simulink model "adc_pdb_trigger_s32k14x"  (Simulink 9.2)
settings: Solver=FixedStepDiscrete  StartTime=0.0  StopTime=10.0  FixedStep=0.1  RelTol=1e-3  EnableMultiTasking=on
InitFcn:
  | mbd_s32k_consistency_checks(bdroot(gcs));
undefined symbols (not defined in the file): LQFP
libraries: mbd_s32k1xx_ec_toolbox x10, simulink x1
Description:
  | This example demonstrates using of ADC module in hardware trigger mode
  | for measuring a signal from AD12 channel (potentiometer) and AD6 channel
  | (temperature)
  | 
  | Validation:
  | - Use adc_pdb_trigger_s32k14x.pmp to validate the ADC conversion
settings Model: Creator=NXP MBDT Team  LastModifiedBy=shivama
settings DataIOCC: ExternalInput=off  InitialState=off  SignalLoggingSaveFormat=Dataset  SaveOutput=off  SignalLogging=off  SaveTime=off
settings OptimizationCC: DefaultParameterBehavior=Inlined  PassReuseOutputArgsAs=Individual arguments  LifeSpan=auto
settings DebuggingCC: SolverPrmCheckMsg=warning  InheritedTsInSrcMsg=none  SingleTaskRateTransMsg=error  ParameterTunabilityLossMsg=error  FcnCallInpInsideContextMsg=error  UnconnectedInputMsg=error  UnconnectedOutputMsg=error  UnconnectedLineMsg=error  AllowSymbolicDim=off  UnknownTsInhSupMsg=error
settings HardwareCC: ProdLargestAtomicInteger=Long  ProdLargestAtomicFloat=Double  ProdEndianess=LittleEndian  ProdHWDeviceType=ARM Compatible->ARM Cortex
settings SFSimCC: MATLABDynamicMemAlloc=off
settings RTWCC: SystemTargetFile=mbd_s32k.tlc  MakeCommand=mbd_s32k_make_rtw COPY_MDLREF_INCLUDES=0  TemplateMakefile=mbd_s32k.tmf  Description=Model Based Design Toolbox S32K14x Code Generation Target  GenerateReport=on  IncludeHyperlinkInReport=on  LaunchReport=on  GenerateTraceInfo=on  GenerateTraceReport=on  GenerateTraceReportSl=on  GenerateTraceReportSf=on  GenerateTraceReportEml=on
settings CodeAppCC: ForceParamTrailComments=on  IgnoreCustomStorageClasses=off  OperatorAnnotations=on  SimulinkDataObjDesc=on  SFDataObjDesc=on  InsertBlockDesc=on  StateflowObjectComments=off
settings STFCustomTargetCC: MultiwordLength=256  ModelReferenceCompliant=off  CombineOutputUpdateFcns=on  ERTCustomFileBanners=on  SupportContinuousTime=off  SupportNonInlinedSFcns=off  RemoveResetFunc=on  MATLABClassNameForMDSCustomization=Simulink.SoftwareTarget.ERTCustomization  GRTInterface=off  SystemTargetFile=mbd_s32k.tlc
settings ERTTargetCC: ModelReferenceCompliant=off  ParMdlRefBuildCompliant=off  CompOptLevelCompliant=off  ConcurrentExecutionCompliant=off  ModelStepFunctionPrototypeControlCompliant=off  CPPClassGenCompliant=off  UseToolchainInfoCompliant=off  InlinedParameterPlacement=NonHierarchical  ERTCustomFileTemplate=example_file_process.tlc

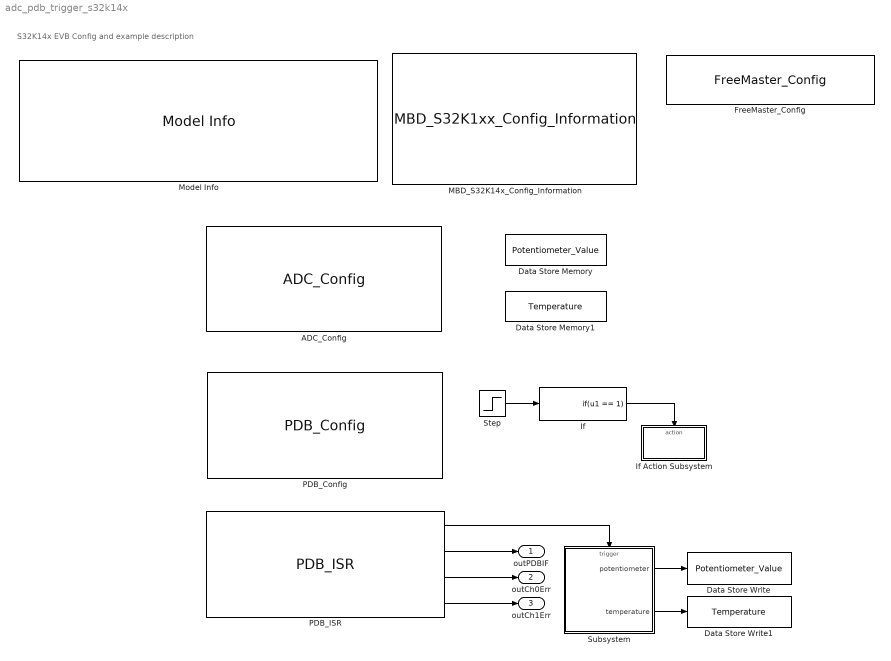
== system adc_pdb_trigger_s32k14x ==
  note: S32K14x EVB Config and example description
  ADC_Config : mbd_s32k1xx_ec_toolbox/Motor Control Blocks/ADC Blocks/ADC_Config  Priority=1  instance=0  mode=12-bit conversion  smplts=29  adiclk=alternate clock 1  adiv=input clock  show_adv_opts=on  pretrgsel=PDB pre-trigger  swpretrg=Disabled  adtrg=hardware  trgsel=PDB output  refsel=Vrefh and Vrefl  supply_monitoring=off  acfe=off  acfgt=off  acren=off  cv1=0  cv2=0  adco=off  avge=off  avgs=4 samples
  Data Store Memory : DataStoreMemory  DataStoreName=Potentiometer_Value  ReadBeforeWriteMsg=warning  WriteAfterWriteMsg=warning  WriteAfterReadMsg=warning  ShowAdditionalParam=off  OutDataTypeStr=uint32
  Data Store Memory1 : DataStoreMemory  DataStoreName=Temperature  ReadBeforeWriteMsg=warning  WriteAfterWriteMsg=warning  WriteAfterReadMsg=warning  ShowAdditionalParam=off  OutDataTypeStr=uint32
  Data Store Write : DataStoreWrite  DataStoreName=Potentiometer_Value
  Data Store Write1 : DataStoreWrite  DataStoreName=Temperature
  FreeMaster_Config : mbd_s32k1xx_ec_toolbox/Utility Blocks/FreeMaster_Config  interface=LPUART1  baudrate=115200  rxd=PTC6: [LPUART1_RX | Receive]  txd=PTC7: [LPUART1_TX | Transmit]  mode=Short Interrupt  isr_prio=15  show_adv_opts=off  use_scope=on  max_scope_vars=8  use_recorder=on  max_rec_vars=8  rec_buff_size=1024  rec_timebase=0 milliseconds  comm_buffer_size_auto=on  comm_buffer_size=255  comm_rqueue_size_default=on  comm_rqueue_size=32
  If : If  IfExpression=u1 == 1  ShowElse=off
  If Action Subsystem : Subsystem  TreatAsAtomicUnit=on
  MBD_S32K14x_Config_Information : mbd_s32k1xx_ec_toolbox/MBD_S32K1xx_Config_Information  mbdt_ver=0  disp_str=|  config_params=[]  mcu_target_name=S32K144  mcu_target_package=100-LQFP  mcu_target_sram_size=64KB  mcu_system_clock_freq=80  mcu_xtal_freq=External 8  mcu_steptick_timer=LPIT Channel 0  mcu_steptick_prio=15  ds_import_enable=on  target_compiler=GCC  target_memory=FLASH  gcc_target_compile_opts=-mcpu=cortex-m4 -mthumb -mfloat-abi=hard -mfpu=fpv4-sp-d16 -O1 -g -gstrict-dwarf  gcc_target_assemble_opts=-mcpu=cortex-m4 -mthumb -mfloat-abi=hard -mfpu=fpv4-sp-d16 -g  gcc_target_link_opts=-mcpu=cortex-m4 -mthumb -mfloat-abi=hard -mfpu=fpv4-sp-d16  gcc_target_default_lcf=on  gcc_target_user_lcf=S32K144_64_flash.ld  ghs_target_compile_opts=-cpu=cortexm4f -thumb -DARM_MATH_CM4 -fpu=vfpv4_d16 -fsingle -Ogeneral -Wundef -Wimplicit-int -Wshadow -Wtrigraphs --no_commons --gnu_asm -gnu99 -gdwarf-2 -G  ghs_target_assemble_opts=-cpu=cortexm4f -fpu=vfpv4_d16  ghs_target_link_opts=-cpu=cortexm4f -thumb -fpu=vfpv4_d16  ghs_target_default_lcf=on  ghs_target_user_lcf=S32K144_64_flash.ld  iar_target_compile_opts=--cpu=Cortex-M4F --thumb --fpu=VFPv4_sp -Ol -e --debug --dlib_config normal  iar_target_assemble_opts=--cpu Cortex-M4F --thumb --fpu VFPv4_sp  iar_target_link_opts=--no_exceptions --vfe --inline  iar_target_default_lcf=on  iar_target_user_lcf=S32K144_64_flash.icf  pil_download_enable=off  rbl_download_enable=on  rbl_start_delay=5000000  rbl_download_interface=OpenSDA  rbl_restart_request=off  rbl_com_port=Custom  rbl_com_port_custom=COM1  pil_download_rate=57600  pil_opensda_drive=D: EVB-S32K144  pil_opensda_drive_custom=D  pil_uart_instance=1  pil_uart_rx=PTC6: [LPUART1_RX | Receive]  pil_uart_tx=PTC7: [LPUART1_TX | Transmit]  FTM_PWM_PcrCheckEnDis=on  FTM_Input_Edge_Inputs_PcrCheckEnDis=on  FTM_Dual_Edge_Inputs_PcrCheckEnDis=on  FTM_Quadrature_Inputs_PcrCheckEnDis=on  FTM_Hall_Sensor_Inputs_PcrCheckEnDis=on  LPTMR_PcrCheckEnDis=on  PIT_PcrCheckEnDis=on  RTC_PcrCheckEnDis=on  FlexCAN_PcrCheckEnDis=on  LIN_PcrCheckEnDis=on  FlexIO_PcrCheckEnDis=on  LPI2C_PcrCheckEnDis=on  LPSPI_PcrCheckEnDis=on  LPUART_PcrCheckEnDis=on  CMP_PcrCheckEnDis=on  GPIO_OutputPcrCheckEnDis=on  GPIO_InputPcrCheckEnDis=on  SBC_PcrCheckEnDis=on  AMMCLIB_PcrCheckEnDis=on  FM_PcrCheckEnDis=on  Profile_PcrCheckEnDis=on  ConfigParams_PcrCheckEnDis=on  ModelRef_PcrCheckEnDis=on  PDB0_PcrCheckEnDis=on  CSEc_PcrCheckEnDis=on  eDMA_PcrCheckEnDis=on  ADC_PcrCheckEnDis=on  WDOG_PcrCheckEnDis=on
      | Target : S32K144-64KB_SRAM
      | Package : 100-pin
      | System clock : 80 MHz
      | XTAL clock : External 8 MHz
      | Compiler : GreenHills Multi
      | Target Type : FLASH
      | Download Code after build : (OpenSDA: F)
      | Step Tick Interrupt Priority : 15
  Model Info : simulink/Model-Wide Utilities/Model Info  Frame=off  DisplayStringWithTags=|  HorizontalTextAlignment=Left  LeftAlignmentValue=0.02
      | Model Name: %<ModelName>
      | 
      | Description: %<Description>
  PDB_Config : mbd_s32k1xx_ec_toolbox/Motor Control Blocks/PDB Blocks/PDB_Config  Priority=1  pdbModule=0  regScCont=Continuous  regScTrgsel=Software  trgMuxSel=FTM2 External Trigger  trgMuxSelPin=PTB5: [TRGMUX_IN0 | Trigger Mux Input]  regModModulus=1200  regScPrescaler=128  regScMult=40  regPoenPoen0=off  regPo0DlyDly1=0  regPo0DlyDly2=0  enable_pdb_init=on  show_adv_opts=off  regCh0C1En0=on  regCh0C1En1=on  regCh0C1En2=off  regCh0C1En3=off  regCh0C1En4=off  regCh0C1En5=off  regCh0C1En6=off  regCh0C1En7=off  regCh0C1Bb0=off  regCh0C1Bb1=off  regCh0C1Bb2=off  regCh0C1Bb3=off  regCh0C1Bb4=off  regCh0C1Bb5=off  regCh0C1Bb6=off  regCh0C1Bb7=off  regCh0C1Tos0=Pre-trigger is in delay mode  regCh0C1Tos1=Pre-trigger is in delay mode  regCh0C1Tos2=Pre-trigger is in delay mode  regCh0C1Tos3=Pre-trigger is in delay mode  regCh0C1Tos4=Pre-trigger is in delay mode  regCh0C1Tos5=Pre-trigger is in delay mode  regCh0C1Tos6=Pre-trigger is in delay mode  regCh0C1Tos7=Pre-trigger is in delay mode  regCh0DlyDly0=120  regCh0DlyDly1=240  regCh0DlyDly2=5000  regCh0DlyDly3=10000  regCh0DlyDly4=0  regCh0DlyDly5=0  regCh0DlyDly6=0  regCh0DlyDly7=0  regCh1C1En0=off  regCh1C1En1=off  regCh1C1En2=off  regCh1C1En3=off  regCh1C1En4=off  regCh1C1En5=off  regCh1C1En6=off  regCh1C1En7=off  regCh1C1Bb0=off  regCh1C1Bb1=off  regCh1C1Bb2=off  regCh1C1Bb3=off  regCh1C1Bb4=off  regCh1C1Bb5=off  regCh1C1Bb6=off  regCh1C1Bb7=off  regCh1C1Tos0=Pre-trigger is in delay mode  regCh1C1Tos1=Pre-trigger is in delay mode  regCh1C1Tos2=Pre-trigger is in delay mode  regCh1C1Tos3=Pre-trigger is in delay mode  regCh1C1Tos4=Pre-trigger is in delay mode  regCh1C1Tos5=Pre-trigger is in delay mode  regCh1C1Tos6=Pre-trigger is in delay mode  regCh1C1Tos7=Pre-trigger is in delay mode  regCh1DlyDly0=0  regCh1DlyDly1=0  regCh1DlyDly2=0  regCh1DlyDly3=0  regCh1DlyDly4=0  regCh1DlyDly5=0  regCh1DlyDly6=0  regCh1DlyDly7=0
  PDB_ISR : mbd_s32k1xx_ec_toolbox/Motor Control Blocks/PDB Blocks/PDB_ISR  Priority=2  pdbModule=0  prioInterrupt=14  regScPdbie=on  regScPdbeie=off  regIdlyIdly=1200
  Step : Step  Time=str2num(get_param(bdroot, 'FixedStep'))  Before=1  After=2
  Subsystem : Subsystem  TreatAsAtomicUnit=on
      settings: RTWSystemCode=Nonreusable function
  outPDBIF : Outport
  outCh0Err : Outport  Port=2
  outCh1Err : Outport  Port=3
  wires:
  Step/1 -> If/1
  If/1 -> If Action Subsystem/Action
  PDB_ISR/2 -> outPDBIF/1
  PDB_ISR/4 -> outCh1Err/1
  PDB_ISR/3 -> outCh0Err/1
  PDB_ISR/1 -> Subsystem/Trigger
  Subsystem/1(potentiometer) -> Data Store Write/1
  Subsystem/2(temperature) -> Data Store Write1/1

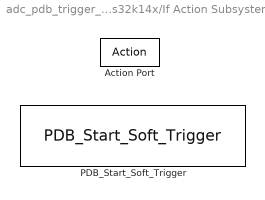
== system adc_pdb_trigger_s32k14x/If Action Subsystem ==
  Action Port : ActionPort
  PDB_Start_Soft_Trigger : mbd_s32k1xx_ec_toolbox/Motor Control Blocks/PDB Blocks/PDB_Start_Soft_Trigger  Priority=9  pdbModule=0

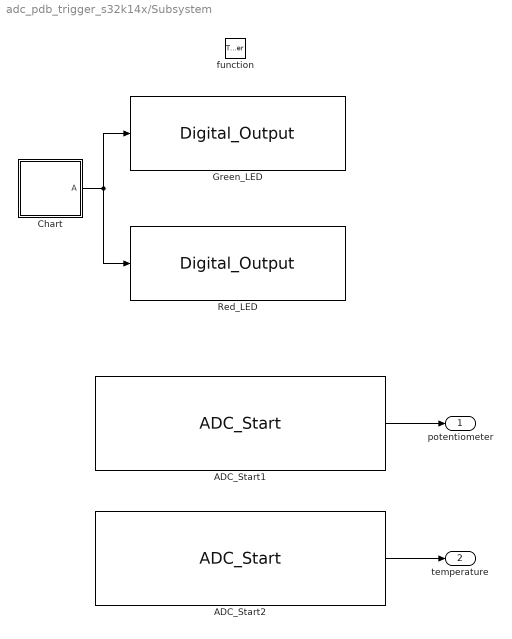
== system adc_pdb_trigger_s32k14x/Subsystem ==
  function : TriggerPort  TriggerType=function-call  VariantControl=Variant
  ADC_Start1 : mbd_s32k1xx_ec_toolbox/Motor Control Blocks/ADC Blocks/ADC_Start  instance=0  adc_r=A  adc_chan=PTC14: [ADC0_SE12 | ADC Single Ended Input]  aien=off  mcuTargetUpdate=on
  ADC_Start2 : mbd_s32k1xx_ec_toolbox/Motor Control Blocks/ADC Blocks/ADC_Start  instance=0  adc_r=B  adc_chan=PTB2: [ADC0_SE6 | ADC Single Ended Input]  aien=off  mcuTargetUpdate=on
  Chart : Stateflow chart  TreatAsAtomicUnit=on
  Green_LED : mbd_s32k1xx_ec_toolbox/GPIO Blocks/Digital_Output  gpio_pin=PTD16: [PTD16 | Port D I/O]  init_val=Low  drive_strength=Low
  Red_LED : mbd_s32k1xx_ec_toolbox/GPIO Blocks/Digital_Output  gpio_pin=PTD15: [PTD15 | Port D I/O]  init_val=Low  drive_strength=Low
  potentiometer : Outport
  temperature : Outport  Port=2
  wires:
  Chart/1(" A") -> Green_LED/1, Red_LED/1
  ADC_Start1/1 -> potentiometer/1
  ADC_Start2/1 -> temperature/1

== stateflow chart Subsystem/Chart ==
  state A
  state A1
  (default) -> A
  A -> A1
  A1 -> A
  data: A output boolean [0..1]
